simulink model "Modelo_asynchronous_machine"  (R2023b)
settings: Solver=ode5  StartTime=0.0  StopTime=0.25  FixedStep=1e-4  RelTol=1e-3
libraries: spsACVoltageSourceLib x9, spsVoltageMeasurementLib x6, spsAsynchronousMachineSIUnitsLib x3, spsGroundLib x3, sps_lib x2, spspowerguiLib x1
settings Model: Creator=HP  LastModifiedBy=HP

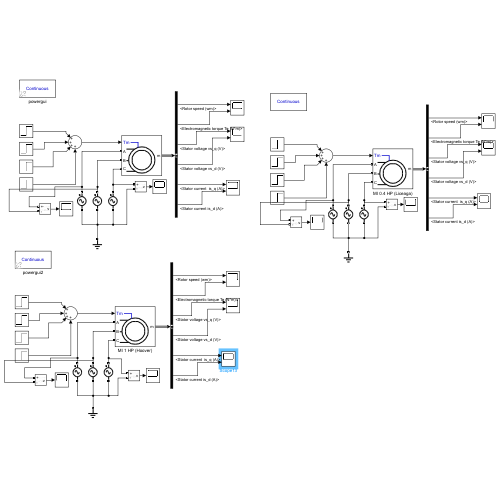
[thumbnail: Simulink's stored preview of the top-level diagram]
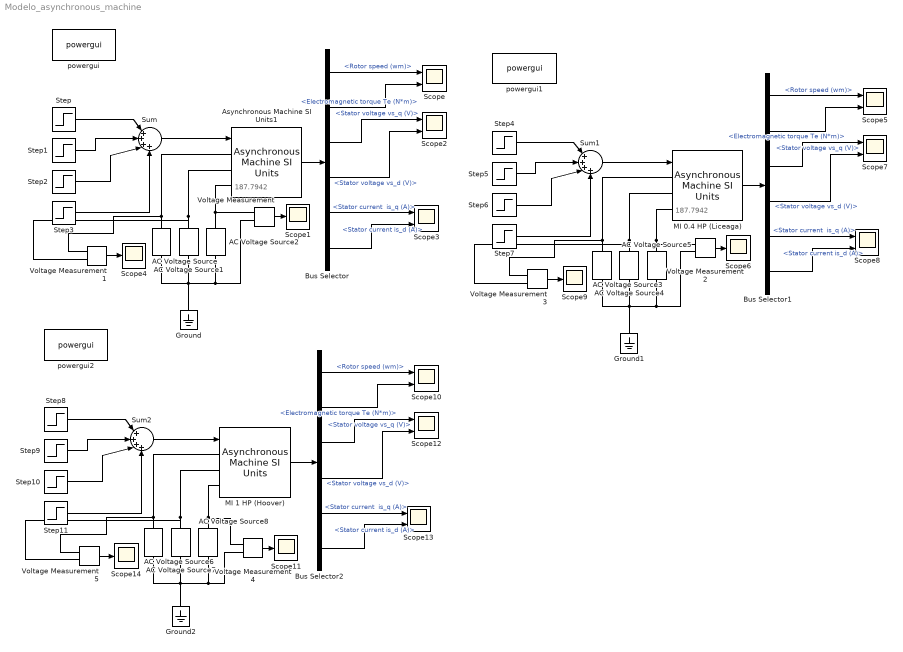
== system Modelo_asynchronous_machine ==
  note: 187.7942
  note: 187.7942
  AC Voltage Source : spsACVoltageSourceLib/AC Voltage Source  Amplitude=375.5884  Phase=0  Frequency=60  SampleTime=0  Measurements=None  BusType=swing  Pref=10e3  Qref=0  Qmin=-inf  Qmax=+inf
  AC Voltage Source1 : spsACVoltageSourceLib/AC Voltage Source  Amplitude=375.5884  Phase=-120  Frequency=60  SampleTime=0  Measurements=None  BusType=swing  Pref=10e3  Qref=0  Qmin=-inf  Qmax=+inf
  AC Voltage Source2 : spsACVoltageSourceLib/AC Voltage Source  Amplitude=375.5884  Phase=120  Frequency=60  SampleTime=0  Measurements=Voltage  BusType=swing  Pref=10e3  Qref=0  Qmin=-inf  Qmax=+inf
  AC Voltage Source3 : spsACVoltageSourceLib/AC Voltage Source  Amplitude=310.268  Phase=0  Frequency=60  SampleTime=0  Measurements=None  BusType=swing  Pref=10e3  Qref=0  Qmin=-inf  Qmax=+inf
  AC Voltage Source4 : spsACVoltageSourceLib/AC Voltage Source  Amplitude=310.268  Phase=-120  Frequency=60  SampleTime=0  Measurements=None  BusType=swing  Pref=10e3  Qref=0  Qmin=-inf  Qmax=+inf
  AC Voltage Source5 : spsACVoltageSourceLib/AC Voltage Source  Amplitude=310.268  Phase=120  Frequency=60  SampleTime=0  Measurements=Voltage  BusType=swing  Pref=10e3  Qref=0  Qmin=-inf  Qmax=+inf
  AC Voltage Source6 : spsACVoltageSourceLib/AC Voltage Source  Amplitude=187.794  Phase=0  Frequency=60  SampleTime=0  Measurements=None  BusType=swing  Pref=10e3  Qref=0  Qmin=-inf  Qmax=+inf
  AC Voltage Source7 : spsACVoltageSourceLib/AC Voltage Source  Amplitude=187.794  Phase=-120  Frequency=60  SampleTime=0  Measurements=None  BusType=swing  Pref=10e3  Qref=0  Qmin=-inf  Qmax=+inf
  AC Voltage Source8 : spsACVoltageSourceLib/AC Voltage Source  Amplitude=187.794  Phase=120  Frequency=60  SampleTime=0  Measurements=Voltage  BusType=swing  Pref=10e3  Qref=0  Qmin=-inf  Qmax=+inf
  Asynchronous Machine SI Units1 : spsAsynchronousMachineSIUnitsLib/Asynchronous Machine SI Units  RotorType=Squirrel-cage  PresetModel="01:  5 HP   460 V 60Hz 1750 RPM"  MechanicalLoad=Torque Tm  ShowDetailedParameters=on  ReferenceFrame=Rotor  Units=SI  MeasurementBus=off  NominalParameters=[3730 460 60]  VoltageRatio=1  Stator=[1.115 0.005974]  Rotor=[1.083 0.005974]  Cage1=[0.4155 0.002066]  Cage2=[0.4168 0.0003495]  Lm=0.2037  Mechanical=[0.02 0.005752 2]  PolePairs=2  InitialConditions=[1 0 0 0 0 0 0 0]  SimulateSaturation=off  Saturation=[14.03593122, 27.81365428, 53.79336849, 72.68890987, 97.98006896, 148.6815601, 215.7428561, 302.9841135, 428.7778367 ; 230, 322, 414, 460, 506, 552, 598, 644, 690]  LoadFlowParameters=1492000  TsPowergui=0  TsBlock=-1  IterativeModel=Trapezoidal non iterative  IterativeDiscreteModel=Trapezoidal non iterative  Pmec=1.492e+006
  Bus Selector : BusSelector  OutputSignals="Mechanical.Rotor speed (wm),Mechanical.Electromagnetic torque Te (N*m),Stator measurements.Stator voltage vs_q (V),Stator measurements.Stator voltage vs_d (V),Stator measurements.Stator current  is_q (A),Stator measurements.Stator current is_d (A)"
  Bus Selector1 : BusSelector  OutputSignals="Mechanical.Rotor speed (wm),Mechanical.Electromagnetic torque Te (N*m),Stator measurements.Stator voltage vs_q (V),Stator measurements.Stator voltage vs_d (V),Stator measurements.Stator current  is_q (A),Stator measurements.Stator current is_d (A)"
  Bus Selector2 : BusSelector  OutputSignals="Mechanical.Rotor speed (wm),Mechanical.Electromagnetic torque Te (N*m),Stator measurements.Stator voltage vs_q (V),Stator measurements.Stator voltage vs_d (V),Stator measurements.Stator current  is_q (A),Stator measurements.Stator current is_d (A)"
  Ground : spsGroundLib/Ground  LConnTagsString=a
  Ground1 : spsGroundLib/Ground  LConnTagsString=a
  Ground2 : spsGroundLib/Ground  LConnTagsString=a
  MI 0.4 HP (Liceaga) : spsAsynchronousMachineSIUnitsLib/Asynchronous Machine SI Units  RotorType=Squirrel-cage  PresetModel=No  MechanicalLoad=Torque Tm  ShowDetailedParameters=on  ReferenceFrame=Stationary  Units=SI  MeasurementBus=off  NominalParameters=[300 380 60]  VoltageRatio=1  Stator=[15.6 0.02]  Rotor=[23.2 0.08]  Cage1=[0.4155 0.002066]  Cage2=[0.4168 0.0003495]  Lm=1.42  Mechanical=[7.11e-4 1.4e-4 1]  PolePairs=2  InitialConditions=[1 0 0 0 0 0 0 0]  SimulateSaturation=off  Saturation=[14.03593122, 27.81365428, 53.79336849, 72.68890987, 97.98006896, 148.6815601, 215.7428561, 302.9841135, 428.7778367 ; 230, 322, 414, 460, 506, 552, 598, 644, 690]  LoadFlowParameters=1492000  TsPowergui=0  TsBlock=-1  IterativeModel=Trapezoidal non iterative  IterativeDiscreteModel=Trapezoidal non iterative  Pmec=1.492e+006
  MI 1 HP (Hoover) : spsAsynchronousMachineSIUnitsLib/Asynchronous Machine SI Units  RotorType=Squirrel-cage  PresetModel=No  MechanicalLoad=Torque Tm  ShowDetailedParameters=on  ReferenceFrame=Stationary  Units=SI  MeasurementBus=off  NominalParameters=[745.7 230 60]  VoltageRatio=1  Stator=[2.516 0.0114]  Rotor=[1.946 0.0077]  Cage1=[0.4155 0.002066]  Cage2=[0.4168 0.0003495]  Lm=0.2226  Mechanical=[0.006276 0.00011 2]  PolePairs=2  InitialConditions=[1 0 0 0 0 0 0 0]  SimulateSaturation=off  Saturation=[14.03593122, 27.81365428, 53.79336849, 72.68890987, 97.98006896, 148.6815601, 215.7428561, 302.9841135, 428.7778367 ; 230, 322, 414, 460, 506, 552, 598, 644, 690]  LoadFlowParameters=1492000  TsPowergui=0  TsBlock=-1  IterativeModel=Trapezoidal non iterative  IterativeDiscreteModel=Trapezoidal non iterative  Pmec=1.492e+006
  Scope{,2..3,5,7..8,10,12..13} (9 alike) : Scope  NumInputPorts=2
  Scope{1,4,6,9,11,14} (6 alike) : Scope
  Step : Step  Time=2.5  After=6.6775  SampleTime=0
  Step1 : Step  Time=5  After=6.6775  SampleTime=0
  Step10 : Step  Time=7.5  After=1.032  SampleTime=0
  Step11 : Step  Time=10  After=1.032  SampleTime=0
  Step2 : Step  Time=7.5  After=6.6775  SampleTime=0
  Step3 : Step  Time=10  After=6.6775  SampleTime=0
  Step4 : Step  Time=2.5  After=0.2076  SampleTime=0
  Step5 : Step  Time=5  After=0.2076  SampleTime=0
  Step6 : Step  Time=7.5  After=0.2076  SampleTime=0
  Step7 : Step  Time=10  After=0.2076  SampleTime=0
  Step8 : Step  Time=2.5  After=1.032  SampleTime=0
  Step9 : Step  Time=5  After=1.032  SampleTime=0
  Sum : Sum  Inputs=|++++
  Sum1 : Sum  Inputs=|++++
  Sum2 : Sum  Inputs=|++++
  Voltage Measurement{,1..5} (6 alike) : spsVoltageMeasurementLib/Voltage Measurement  PhasorSimulation=off  OutputType=Complex  PSBequivalent=0
  powergui : sps_lib/powergui  Priority=1  SimulationMode=Continuous  SampleTime=50e-6  frequency=60  Iterations=50  frequencyindice=60  Pbase=100e6  ErrMax=1e-4  UnitsV=kV  UnitsW=MW  buscounter=0  FunctionMessages=off  echomessages=off  EnableUseOfTLC=off  CurrentSourceSwitches=off  DisableSnubberDevices=off  DisableRonSwitches=off  DisableVfSwitches=off  DisplayEquations=off  AutomaticDiscreteSolvers=off  SolverType=Tustin/Backward Euler (TBE)  Interpol=off  ExternalGateDelay=off  methode=off  Ts=100  x0status=blocks  SPID=on  SwTol=0  HookPort=off  NonlinearTolerance=1e-4  nMaxIteration=100  ContinueOnMaxIteration=off  RestoreLinks=warning  ResistiveCurrentMeasurement=off  Frange=[0:2:500]  Ylog=off  Xlog=on  ShowGrid=off  save=off  variable=ZData  structure=0  ZoomFFT=off  StartTime=0.0  cycles=1  DisplayStyle=1  fundamental=60  FreqAxis=off  MaxFrequency=1000  frequencyindicesteady=1  RmsSteady=1  display=off
  powergui1 : spspowerguiLib/powergui  Priority=1  SimulationMode=Continuous  SampleTime=50e-6  frequency=60  Iterations=50  frequencyindice=60  Pbase=100e6  ErrMax=1e-4  UnitsV=kV  UnitsW=MW  buscounter=0  FunctionMessages=off  echomessages=off  EnableUseOfTLC=off  CurrentSourceSwitches=off  DisableSnubberDevices=off  DisableRonSwitches=off  DisableVfSwitches=off  DisplayEquations=off  AutomaticDiscreteSolvers=off  SolverType=Tustin/Backward Euler (TBE)  Interpol=off  ExternalGateDelay=off  methode=off  Ts=100  x0status=blocks  SPID=on  SwTol=0  HookPort=off  NonlinearTolerance=1e-4  nMaxIteration=100  ContinueOnMaxIteration=off  RestoreLinks=warning  ResistiveCurrentMeasurement=off  Frange=[0:2:500]  Ylog=off  Xlog=on  ShowGrid=off  save=off  variable=ZData  structure=0  ZoomFFT=off  StartTime=0.0  cycles=1  DisplayStyle=1  fundamental=60  FreqAxis=off  MaxFrequency=1000  frequencyindicesteady=1  RmsSteady=1  display=off
  powergui2 : sps_lib/powergui  Priority=1  SimulationMode=Continuous  SampleTime=50e-6  frequency=60  Iterations=50  frequencyindice=60  Pbase=100e6  ErrMax=1e-4  UnitsV=kV  UnitsW=MW  buscounter=0  FunctionMessages=off  echomessages=off  EnableUseOfTLC=off  CurrentSourceSwitches=off  DisableSnubberDevices=off  DisableRonSwitches=off  DisableVfSwitches=off  DisplayEquations=off  AutomaticDiscreteSolvers=off  SolverType=Tustin/Backward Euler (TBE)  Interpol=off  ExternalGateDelay=off  methode=off  Ts=100  x0status=blocks  SPID=on  SwTol=0  HookPort=off  NonlinearTolerance=1e-4  nMaxIteration=100  ContinueOnMaxIteration=off  RestoreLinks=warning  ResistiveCurrentMeasurement=off  Frange=[0:2:500]  Ylog=off  Xlog=on  ShowGrid=off  save=off  variable=ZData  structure=0  ZoomFFT=off  StartTime=0.0  cycles=1  DisplayStyle=1  fundamental=60  FreqAxis=off  MaxFrequency=1000  frequencyindicesteady=1  RmsSteady=1  display=off
  wires:
  Asynchronous Machine SI Units1/1 -> Bus Selector/1
  Bus Selector/2 -> Scope/2  "<Electromagnetic torque Te (N*m)>"
  Bus Selector/1 -> Scope/1  "<Rotor speed (wm)>"
  Step/1 -> Sum/1
  Step1/1 -> Sum/2
  Step2/1 -> Sum/3
  Step3/1 -> Sum/4
  Voltage Measurement/1 -> Scope1/1
  Bus Selector/3 -> Scope2/1  "<Stator voltage vs_q (V)>"
  Bus Selector/4 -> Scope2/2  "<Stator voltage vs_d (V)>"
  Sum/1 -> Asynchronous Machine SI Units1/1
  Bus Selector/5 -> Scope3/1  "<Stator current  is_q (A)>"
  Bus Selector/6 -> Scope3/2  "<Stator current is_d (A)>"
  Voltage Measurement1/1 -> Scope4/1
  MI 0.4 HP (Liceaga)/1 -> Bus Selector1/1
  Voltage Measurement3/1 -> Scope9/1
  Bus Selector1/2 -> Scope5/2  "<Electromagnetic torque Te (N*m)>"
  Bus Selector1/6 -> Scope8/2  "<Stator current is_d (A)>"
  Bus Selector1/4 -> Scope7/2  "<Stator voltage vs_d (V)>"
  Step7/1 -> Sum1/4
  Voltage Measurement2/1 -> Scope6/1
  Step5/1 -> Sum1/2
  Bus Selector1/3 -> Scope7/1  "<Stator voltage vs_q (V)>"
  Sum1/1 -> MI 0.4 HP (Liceaga)/1
  Bus Selector1/5 -> Scope8/1  "<Stator current  is_q (A)>"
  Step4/1 -> Sum1/1
  Step6/1 -> Sum1/3
  Bus Selector1/1 -> Scope5/1  "<Rotor speed (wm)>"
  Bus Selector2/2 -> Scope10/2  "<Electromagnetic torque Te (N*m)>"
  Voltage Measurement5/1 -> Scope14/1
  Sum2/1 -> MI 1 HP (Hoover)/1
  Bus Selector2/4 -> Scope12/2  "<Stator voltage vs_d (V)>"
  Voltage Measurement4/1 -> Scope11/1
  Step11/1 -> Sum2/4
  Bus Selector2/6 -> Scope13/2  "<Stator current is_d (A)>"
  Bus Selector2/5 -> Scope13/1  "<Stator current  is_q (A)>"
  Step8/1 -> Sum2/1
  Step9/1 -> Sum2/2
  Step10/1 -> Sum2/3
  Bus Selector2/1 -> Scope10/1  "<Rotor speed (wm)>"
  MI 1 HP (Hoover)/1 -> Bus Selector2/1
  Bus Selector2/3 -> Scope12/1  "<Stator voltage vs_q (V)>"
  connections:
  Ground/LConn1 -- AC Voltage Source/LConn1 -- AC Voltage Source1/LConn1 -- Voltage Measurement/LConn2 -- AC Voltage Source2/LConn1
  AC Voltage Source2/RConn1 -- Asynchronous Machine SI Units1/LConn3 -- Voltage Measurement/LConn1
  Asynchronous Machine SI Units1/LConn2 -- Voltage Measurement1/LConn2 -- AC Voltage Source1/RConn1
  Asynchronous Machine SI Units1/LConn1 -- Voltage Measurement1/LConn1 -- AC Voltage Source/RConn1
  AC Voltage Source3/RConn1 -- MI 0.4 HP (Liceaga)/LConn1 -- Voltage Measurement3/LConn1
  Voltage Measurement2/LConn2 -- AC Voltage Source3/LConn1 -- Ground1/LConn1 -- AC Voltage Source4/LConn1 -- AC Voltage Source5/LConn1
  Voltage Measurement2/LConn1 -- MI 0.4 HP (Liceaga)/LConn3 -- AC Voltage Source5/RConn1
  AC Voltage Source4/RConn1 -- MI 0.4 HP (Liceaga)/LConn2 -- Voltage Measurement3/LConn2
  Voltage Measurement4/LConn2 -- AC Voltage Source6/LConn1 -- Ground2/LConn1 -- AC Voltage Source7/LConn1 -- AC Voltage Source8/LConn1
  AC Voltage Source6/RConn1 -- MI 1 HP (Hoover)/LConn1 -- Voltage Measurement5/LConn1
  AC Voltage Source7/RConn1 -- MI 1 HP (Hoover)/LConn2 -- Voltage Measurement5/LConn2
  Voltage Measurement4/LConn1 -- MI 1 HP (Hoover)/LConn3 -- AC Voltage Source8/RConn1
